simulink model "thrusterTest"  (R2013a)
settings: Solver=ode45  StartTime=0.0  StopTime=10.0  RelTol=1e-3
undefined symbols (not defined in the file or in its folder): rho, thruster
settings Model: Creator=torstebo  LastModifiedBy=torstebo
settings DataIOCC: InspectSignalLogs=on

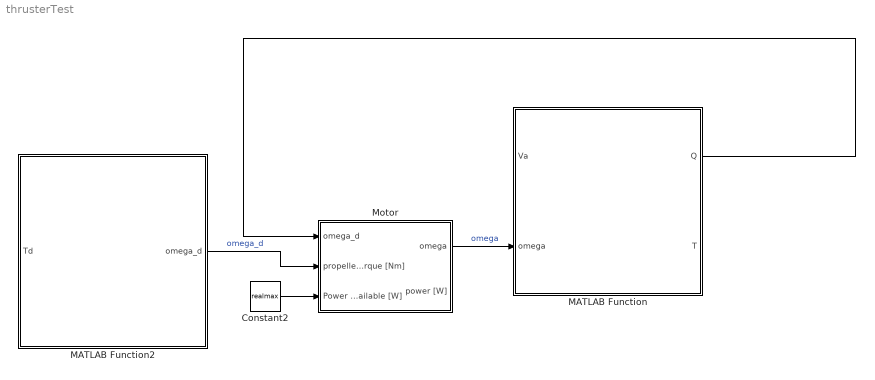
== system thrusterTest ==
  Constant2 : Constant  Value=realmax
  MATLAB Function : MATLAB Function  TreatAsAtomicUnit=on
  MATLAB Function2 : MATLAB Function  TreatAsAtomicUnit=on
  Motor : Subsystem
  wires:
  MATLAB Function2/1(omega_d) -> Motor/2(propeller torque [Nm])  "omega_d"
  Motor/1(omega) -> MATLAB Function/2(omega)  "omega"
  MATLAB Function/1(Q) -> Motor/1(omega_d)
  Constant2/1 -> Motor/3(Power Available [W])

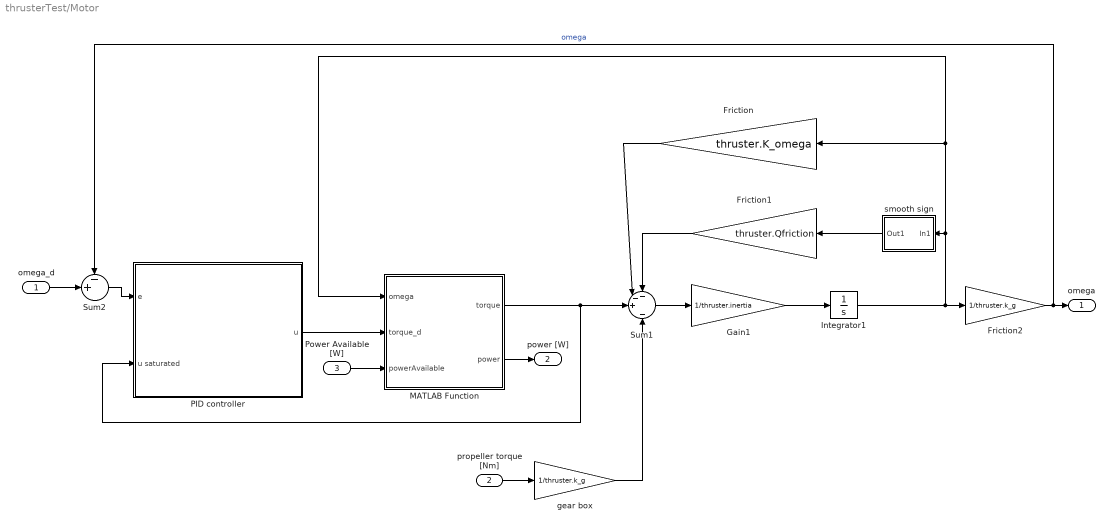
== system thrusterTest/Motor ==
  omega_d : Inport
  propeller torque [Nm] : Inport  Port=2
  Power Available [W] : Inport  Port=3
  Friction : Gain  Gain=thruster.K_omega
  Friction1 : Gain  Gain=thruster.Qfriction
  Friction2 : Gain  Gain=1/thruster.k_g
  Gain1 : Gain  Gain=1/thruster.inertia
  Integrator1 : Integrator  InitialCondition=thruster.motor.omega0
  MATLAB Function : MATLAB Function  TreatAsAtomicUnit=on
  PID controller : Subsystem
  Sum1 : Sum  Inputs=--+|-
  Sum2 : Sum  Inputs=-+|
  gear box : Gain  Gain=1/thruster.k_g
  smooth sign : Subsystem
  omega : Outport
  power [W] : Outport  Port=2
  wires:
  Integrator1/1 -> MATLAB Function/1(omega), Friction/1, smooth sign/1(In1), Friction2/1
  Sum1/1 -> Gain1/1
  Gain1/1 -> Integrator1/1
  gear box/1 -> Sum1/4
  Friction/1 -> Sum1/2
  MATLAB Function/1(torque) -> PID controller/2(u saturated), Sum1/3
  MATLAB Function/2(power) -> power [W]/1
  smooth sign/1(Out1) -> Friction1/1
  Friction1/1 -> Sum1/1
  Friction2/1 -> Sum2/1, omega/1  "omega"
  propeller torque [Nm]/1 -> gear box/1
  omega_d/1 -> Sum2/2
  Sum2/1 -> PID controller/1(e)
  PID controller/1(u) -> MATLAB Function/2(torque_d)
  Power Available [W]/1 -> MATLAB Function/3(powerAvailable)

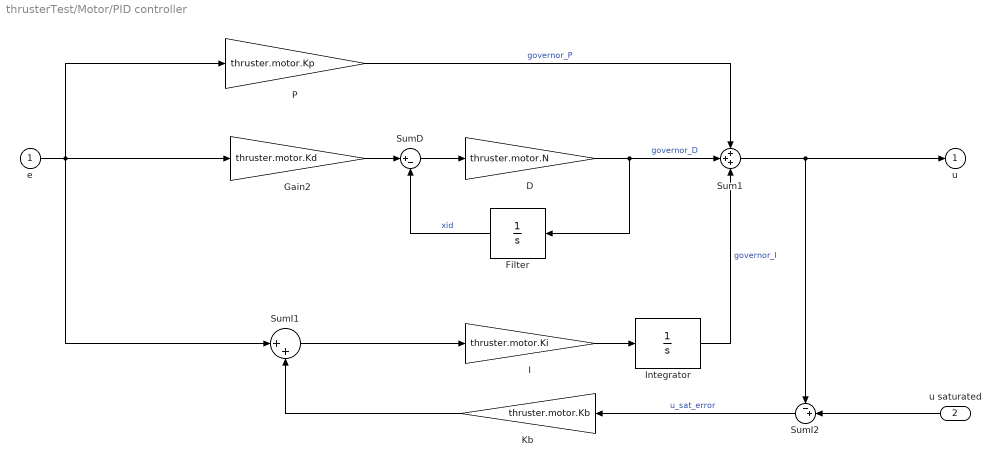
== system thrusterTest/Motor/PID controller ==
  e : Inport  PortDimensions=1
  u saturated : Inport  Port=2  PortDimensions=1
  D : Gain  DisableCoverage=on  Gain=thruster.motor.N
  Filter : Integrator  DisableCoverage=on
  Gain2 : Gain  Gain=thruster.motor.Kd
  I : Gain  Gain=thruster.motor.Ki
  Integrator : Integrator  DisableCoverage=on  InitialCondition=thruster.motor.torque0
  Kb : Gain  DisableCoverage=on  Gain=thruster.motor.Kb  ParamDataTypeStr=Inherit: Inherit from 'Gain'
  P : Gain  Gain=thruster.motor.Kp
  Sum1 : Sum  Inputs=+++
  SumD : Sum  DisableCoverage=on  Inputs=|+-
  SumI1 : Sum  DisableCoverage=on  Inputs=|++
  SumI2 : Sum  DisableCoverage=on  Inputs=-+|
  u : Outport  PortDimensions=1  InitialOutput=0
  wires:
  I/1 -> Integrator/1
  SumI1/1 -> I/1
  u saturated/1 -> SumI2/2
  Kb/1 -> SumI1/2
  SumI2/1 -> Kb/1  "u_sat_error"
  Gain2/1 -> SumD/1
  SumD/1 -> D/1
  Filter/1 -> SumD/2  "xid"
  Sum1/1 -> u/1, SumI2/1
  P/1 -> Sum1/1  "governor_P"
  e/1 -> Gain2/1, SumI1/1, P/1
  D/1 -> Filter/1, Sum1/2  "governor_D"
  Integrator/1 -> Sum1/3  "governor_I"

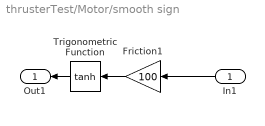
== system thrusterTest/Motor/smooth sign ==
  In1 : Inport
  Friction1 : Gain  Gain=100
  Trigonometric Function : Trigonometry  Operator=tanh
  Out1 : Outport
  wires:
  Friction1/1 -> Trigonometric Function/1
  Trigonometric Function/1 -> Out1/1
  In1/1 -> Friction1/1

== matlab function thrusterTest/MATLAB Function2 ==
  data: Td input; omega_d output; thruster parameter; rho parameter
function omega_d  = propeller(Td,thruster,rho)
%#codegen
omega_d = findDesiredPropellerSpeed(Td,thruster,rho);

== matlab function thrusterTest/MATLAB Function ==
  data: Q output; Va input; omega input; T output; thruster parameter; rho parameter
function [Q,T] = propeller(Va,omega,thruster,rho)
%#codegen
beta = atan2(Va,0.7*pi*omega*thruster.radius);
Ct = 0;
Cq = 0;
for i = 1:length(thruster.AT)
    Ct = Ct + thruster.AT(i)*cos(beta*(i-1))+thruster.BT(i)*sin(beta*(i-1));
    Cq = Cq + thruster.AQ(i)*cos(beta*(i-1))+thruster.BQ(i)*sin(beta*(i-1));
end
V07_2 = Va^2+(0.7*omega*thruster.radius)^2;
T = Ct*.5*rho*V07_2*pi*thruster.radius^2;
Q = Cq*.5*rho*V07_2*pi*2*thruster.radius^3;

== matlab function thrusterTest/Motor/MATLAB Function ==
  data: omega input; torque_d input; torque output; thruster parameter; power output; powerAvailable input
function [torque, power] = saturation(omega,torque_d,thruster,powerAvailable)
%#codegen
% check for inverse power
if (omega*torque_d<0)
    torque = 0;
    power = 0;
    return
end

% check maximum torque
torque_d = sign(torque_d)*min(thruster.Qmax,abs(torque_d));

% check maximum power (has checked for inverse power)
pMax = min(thruster.Pmax,powerAvailable);
if (omega*torque_d>pMax)
    torque_d = torque_d*(pMax/omega*torque_d);
end

torque = torque_d;
power = torque*omega;
